simulink model "can8auto"  (R2018a)
settings: Solver=VariableStepAuto  StartTime=0.0  StopTime=5000  RelTol=1e-3
libraries: commcrc2 x20, simulink x20, simulink_extras x5, dspswit3 x5
(part 7 of 7)

== matlab function can8auto/CAN MASTER/MATLAB Function ==
  data: parallel input; serial output size=1; current_index input size=1; next_index output size=1; state input; endTX output
  events: trigger input RISING_EDGE_EVENT
function [serial,next_index,endTX] = parallelToSerial(parallel,current_index, state)
    size_parallel = size(parallel);
    size_parallel = size_parallel(2);
    endTX = 0;
    serial = 1;
    next_index = 1;
    if current_index < size_parallel && (state == 2 || state == 3)
        serial = parallel(current_index+1);
        next_index = current_index + 1;
        return
    end
    if current_index == size_parallel && (state == 2 || state == 3)
        endTX = 1;
    end
end

== matlab function can8auto/SDO NODO CAN/CAN NODE/SDO Frame generator/BitStuffing/MATLAB Function ==
  data: u input; b output
function b = fcn(u)
a = u;
b = zeros(1,floor(length(a)+length(a)/5));
k = 0;
count2 = 1;
i = 1;
n = length(a);
count = 1;
j = 1;
while i < n
    if a(i) == 1
        b(j) = a(i);
        while a(i+1) == 1 && i+1 < n && count < 5
            j = j+1;
            b(j) = a(i+1);
            count = count + 1;
            count2 = count;
            if count == 5
                j = j+1;
                b(j) = 0;
            end
            i = i+1;
        end
        
    else
        b(j) = a(i);
    end
    
    if a(i) == 0
    if a(i) == 0
        b(j) = a(i);
        while a(i+1) == 0 && i+1 < n && count < 5
            j = j+1;
            b(j) = a(i+1);
            count = count + 1;
            count2 = count;
            if count == 5
                j = j+1;
                b(j) = 1;
            end
            i = i+1;
        end
        
    else
        b(j) = a(i);
    end
    end
    
    i = i+1;
    j = j+1;
    count = 1;
end
if i == n && a(i) == 1 && count2 == 4
    b(j) = a(i);
    b(j+1) = 0;
else
    b(j) = a(i);
end

if i == n && a(i) == 0 && count2 == 4
    b(j) = a(i);
    b(j+1) = 1;
else
    b(j) = a(i);
end

== stateflow chart can8auto/SDO NODO CAN/SlaveSDO ==
  state BootUp
    entry: mode = 0;
  state NormalOp
    entry: mode = 2;
  (default) -> BootUp
  NormalOp -> BootUp : [rst == 1]
  BootUp -> NormalOp : [SDO == 1 && EndTX == 1 && TotTX == 2]
  data: rst input; SDO input; TotTX input; EndTX input; mode output

== matlab function can8auto/SYNC PRODUCER/CAN NODE/Bootup Frame generator/BitStuffing/MATLAB Function ==
  data: u input; b output
function b = fcn(u)
a = u;
b = zeros(1,floor(length(a)+length(a)/5));
k = 0;
count2 = 1;
i = 1;
n = length(a);
count = 1;
j = 1;
while i < n
    if a(i) == 1
        b(j) = a(i);
        while a(i+1) == 1 && i+1 < n && count < 5
            j = j+1;
            b(j) = a(i+1);
            count = count + 1;
            count2 = count;
            if count == 5
                j = j+1;
                b(j) = 0;
            end
            i = i+1;
        end
        
    else
        b(j) = a(i);
    end
    
    if a(i) == 0
    if a(i) == 0
        b(j) = a(i);
        while a(i+1) == 0 && i+1 < n && count < 5
            j = j+1;
            b(j) = a(i+1);
            count = count + 1;
            count2 = count;
            if count == 5
                j = j+1;
                b(j) = 1;
            end
            i = i+1;
        end
        
    else
        b(j) = a(i);
    end
    end
    
    i = i+1;
    j = j+1;
    count = 1;
end
if i == n && a(i) == 1 && count2 == 4
    b(j) = a(i);
    b(j+1) = 0;
else
    b(j) = a(i);
end

if i == n && a(i) == 0 && count2 == 4
    b(j) = a(i);
    b(j+1) = 1;
else
    b(j) = a(i);
end

== matlab function can8auto/SDO NODO CAN/CAN NODE/SDO Frame generator/MUX/MATLAB Function ==
  data: index input; result output size=[1 64]; u1 input
function result  = mux(index, u1)
%#codegen
%
% Insert zeros between elements

result = zeros(1,64);
switch index
    case 0
        result = u1(1:64);
    case 1
        result = u1(65:128);
    case 2
        result = u1(129:192);
    otherwise
        result = u1(193:256);
end

== matlab function can8auto/SYNC PRODUCER/MATLAB Function ==
  data: u input size=1; y output size=1
function y = equals4(u)
    if u == 4
        y = 1;
    else
        y = 0;
    end
end

== matlab function can8auto/SYNC PRODUCER/CAN NODE/Frame MUX/MATLAB Function2 ==
  data: mode input; result output size=[1 200]; u1 input; size input
function result = MUX_lv2(mode, u1, size)
%#codegen
%
% Insert zeros between elements

switch mode
    case 0
        result = u1(1 : size(1));
    case 1
        result = u1(size(1)+1 : size(1)+size(2));
    case 2
        result = u1(size(1)+size(2)+1 : size(1)+size(2)+size(3));
    case 3
        result = u1(size(1)+size(2)+size(3)+1 : size(1)+size(2)+size(3)+size(4));
    otherwise
        result = u1(size(1)+size(2)+size(3)+size(4)+1 : size(1)+size(2)+size(3)+size(4)+size(5));
end

== stateflow chart can8auto/CAN MASTER/Master ==
  state BootUp
    entry: sigOut = 0;
  state NMT
    entry: PDO = 1;
    entry: SDO = 1;
    entry: sigOut = 1;
  state NormalOp
    entry: sigOut = 2;
  (default) -> BootUp
  BootUp -> NMT : [EndTX == 1 && totalTX == 2]
  NormalOp -> BootUp : [rst == 1]
  NMT -> NormalOp : [EndTX == 1 && totalTX == 3]
  data: rst input; SDO output; PDO output; sigOut output; EndTX input; totalTX input

== matlab function can8auto/CAN MASTER/MATLAB Function1 ==
  data: u input size=1; y output size=1
function y = fcn(u)
if u == 1
    y = true;
else
    y = false;
end

== matlab function can8auto/SDO NODO CAN/CAN NODE/SYNC Frame Generator/BitStuffing/MATLAB Function ==
  data: u input; b output
function b = fcn(u)
a = u;
b = zeros(1,floor(length(a)+length(a)/5));
k = 0;
count2 = 1;
i = 1;
n = length(a);
count = 1;
j = 1;
while i < n
    if a(i) == 1
        b(j) = a(i);
        while a(i+1) == 1 && i+1 < n && count < 5
            j = j+1;
            b(j) = a(i+1);
            count = count + 1;
            count2 = count;
            if count == 5
                j = j+1;
                b(j) = 0;
            end
            i = i+1;
        end
        
    else
        b(j) = a(i);
    end
    
    if a(i) == 0
    if a(i) == 0
        b(j) = a(i);
        while a(i+1) == 0 && i+1 < n && count < 5
            j = j+1;
            b(j) = a(i+1);
            count = count + 1;
            count2 = count;
            if count == 5
                j = j+1;
                b(j) = 1;
            end
            i = i+1;
        end
        
    else
        b(j) = a(i);
    end
    end
    
    i = i+1;
    j = j+1;
    count = 1;
end
if i == n && a(i) == 1 && count2 == 4
    b(j) = a(i);
    b(j+1) = 0;
else
    b(j) = a(i);
end

if i == n && a(i) == 0 && count2 == 4
    b(j) = a(i);
    b(j+1) = 1;
else
    b(j) = a(i);
end

== stateflow chart can8auto/SDO NODO CAN/Chart ==
  state NoTX
    entry: state = 0;
  state SenseBus
    entry: state = 1;
  state TXcompleated
    entry: state = 4;
  state TX
    entry: state = 2;
  NoTX -> NoTX [order 2] : [Frame == 0]
  SenseBus -> SenseBus [order 1] : [Free == 0 || EndTX == 1]
  (default) -> NoTX
  TXcompleated -> NoTX [order 1] : [Frame == 0]
  NoTX -> SenseBus [order 1] : [Frame  > 0]
  TX -> SenseBus [order 2] : [Error == 1]
  TXcompleated -> SenseBus [order 2] : [Frame  > 0]
  SenseBus -> TX [order 2] : [Free == 1]
  TX -> TXcompleated [order 1] : [EndTX == 1]
  TX -> TX [order 3]
  data: Free input; Error input; Frame input; EndTX input; state output

== matlab function can8auto/SDO NODO CAN/MATLAB Function ==
  data: parallel input; serial output size=1; current_index input size=1; next_index output size=1; state input; endTX output
  events: trigger input RISING_EDGE_EVENT
function [serial,next_index,endTX] = parallelToSerial(parallel,current_index, state)
    size_parallel = size(parallel);
    size_parallel = size_parallel(2);
    endTX = 0;
    serial = 1;
    next_index = 1;
    if current_index < size_parallel && (state == 2 || state == 3)
        serial = parallel(current_index+1);
        next_index = current_index + 1;
        return
    end
    if current_index == size_parallel && (state == 2 || state == 3)
        endTX = 1;
    end
end

== matlab function can8auto/SDO NODO CAN/MATLAB Function1 ==
  data: u input size=1; y output size=1
function y = fcn(u)
if u == 1
    y = true;
else
    y = false;
end

== matlab function can8auto/SDO NODO CAN/Sensing/MATLAB Function ==
  data: BusState input; free output; clock input; count input; count output
  events: trigger input RISING_EDGE_EVENT
function [free, count] = fcn(BusState, clock, count)
if clock
    if BusState
        count = count + 1;
    else
        count = 0;
    end
end
if count >= 20
    free = 1;
else
    free = 0;
end

== matlab function can8auto/CAN MASTER/Sensing/MATLAB Function ==
  data: BusState input; free output; clock input; count input; count output
  events: trigger input RISING_EDGE_EVENT
function [free, count] = fcn(BusState, clock, count)
if clock
    if BusState
        count = count + 1;
    else
        count = 0;
    end
end
if count >= 20
    free = 1;
else
    free = 0;
end

== stateflow chart can8auto/PDO NODO CAN /SlavePDO ==
  state BootUp
    entry: mode = 0;
  state Normal
    entry: mode = 3;
  (default) -> BootUp
  Normal -> BootUp : [rst == 1]
  BootUp -> Normal : [PDO == 1 && EndTX == 1]
  data: rst input; PDO input; EndTX input; mode output

== matlab function can8auto/SYNC PRODUCER/CAN NODE/NMT Frame generator/BitStuffing/MATLAB Function ==
  data: u input; b output
function b = fcn(u)
a = u;
b = zeros(1,floor(length(a)+length(a)/5));
k = 0;
count2 = 1;
i = 1;
n = length(a);
count = 1;
j = 1;
while i < n
    if a(i) == 1
        b(j) = a(i);
        while a(i+1) == 1 && i+1 < n && count < 5
            j = j+1;
            b(j) = a(i+1);
            count = count + 1;
            count2 = count;
            if count == 5
                j = j+1;
                b(j) = 0;
            end
            i = i+1;
        end
        
    else
        b(j) = a(i);
    end
    
    if a(i) == 0
    if a(i) == 0
        b(j) = a(i);
        while a(i+1) == 0 && i+1 < n && count < 5
            j = j+1;
            b(j) = a(i+1);
            count = count + 1;
            count2 = count;
            if count == 5
                j = j+1;
                b(j) = 1;
            end
            i = i+1;
        end
        
    else
        b(j) = a(i);
    end
    end
    
    i = i+1;
    j = j+1;
    count = 1;
end
if i == n && a(i) == 1 && count2 == 4
    b(j) = a(i);
    b(j+1) = 0;
else
    b(j) = a(i);
end

if i == n && a(i) == 0 && count2 == 4
    b(j) = a(i);
    b(j+1) = 1;
else
    b(j) = a(i);
end

== matlab function can8auto/SYNC PRODUCER/CAN NODE/SDO Frame generator/BitStuffing/MATLAB Function ==
  data: u input; b output
function b = fcn(u)
a = u;
b = zeros(1,floor(length(a)+length(a)/5));
k = 0;
count2 = 1;
i = 1;
n = length(a);
count = 1;
j = 1;
while i < n
    if a(i) == 1
        b(j) = a(i);
        while a(i+1) == 1 && i+1 < n && count < 5
            j = j+1;
            b(j) = a(i+1);
            count = count + 1;
            count2 = count;
            if count == 5
                j = j+1;
                b(j) = 0;
            end
            i = i+1;
        end
        
    else
        b(j) = a(i);
    end
    
    if a(i) == 0
    if a(i) == 0
        b(j) = a(i);
        while a(i+1) == 0 && i+1 < n && count < 5
            j = j+1;
            b(j) = a(i+1);
            count = count + 1;
            count2 = count;
            if count == 5
                j = j+1;
                b(j) = 1;
            end
            i = i+1;
        end
        
    else
        b(j) = a(i);
    end
    end
    
    i = i+1;
    j = j+1;
    count = 1;
end
if i == n && a(i) == 1 && count2 == 4
    b(j) = a(i);
    b(j+1) = 0;
else
    b(j) = a(i);
end

if i == n && a(i) == 0 && count2 == 4
    b(j) = a(i);
    b(j+1) = 1;
else
    b(j) = a(i);
end

== matlab function can8auto/PDO NODO CAN /CAN NODE/Bootup Frame generator/BitStuffing/MATLAB Function ==
  data: u input; b output
function b = fcn(u)
a = u;
b = zeros(1,floor(length(a)+length(a)/5));
k = 0;
count2 = 1;
i = 1;
n = length(a);
count = 1;
j = 1;
while i < n
    if a(i) == 1
        b(j) = a(i);
        while a(i+1) == 1 && i+1 < n && count < 5
            j = j+1;
            b(j) = a(i+1);
            count = count + 1;
            count2 = count;
            if count == 5
                j = j+1;
                b(j) = 0;
            end
            i = i+1;
        end
        
    else
        b(j) = a(i);
    end
    
    if a(i) == 0
    if a(i) == 0
        b(j) = a(i);
        while a(i+1) == 0 && i+1 < n && count < 5
            j = j+1;
            b(j) = a(i+1);
            count = count + 1;
            count2 = count;
            if count == 5
                j = j+1;
                b(j) = 1;
            end
            i = i+1;
        end
        
    else
        b(j) = a(i);
    end
    end
    
    i = i+1;
    j = j+1;
    count = 1;
end
if i == n && a(i) == 1 && count2 == 4
    b(j) = a(i);
    b(j+1) = 0;
else
    b(j) = a(i);
end

if i == n && a(i) == 0 && count2 == 4
    b(j) = a(i);
    b(j+1) = 1;
else
    b(j) = a(i);
end

== matlab function can8auto/SYNC PRODUCER/CAN NODE/SDO Frame generator/MUX/MATLAB Function ==
  data: index input; result output size=[1 64]; u1 input
function result  = mux(index, u1)
%#codegen
%
% Insert zeros between elements

result = zeros(1,64);
switch index
    case 0
        result = u1(1:64);
    case 1
        result = u1(65:128);
    case 2
        result = u1(129:192);
    otherwise
        result = u1(193:256);
end

== matlab function can8auto/PDO NODO CAN /CAN NODE/Frame MUX/MATLAB Function2 ==
  data: mode input; result output size=[1 200]; u1 input; size input
function result = MUX_lv2(mode, u1, size)
%#codegen
%
% Insert zeros between elements

switch mode
    case 0
        result = u1(1 : size(1));
    case 1
        result = u1(size(1)+1 : size(1)+size(2));
    case 2
        result = u1(size(1)+size(2)+1 : size(1)+size(2)+size(3));
    case 3
        result = u1(size(1)+size(2)+size(3)+1 : size(1)+size(2)+size(3)+size(4));
    otherwise
        result = u1(size(1)+size(2)+size(3)+size(4)+1 : size(1)+size(2)+size(3)+size(4)+size(5));
end

== matlab function can8auto/PDO NODO CAN /CAN NODE/NMT Frame generator/BitStuffing/MATLAB Function ==
  data: u input; b output
function b = fcn(u)
a = u;
b = zeros(1,floor(length(a)+length(a)/5));
k = 0;
count2 = 1;
i = 1;
n = length(a);
count = 1;
j = 1;
while i < n
    if a(i) == 1
        b(j) = a(i);
        while a(i+1) == 1 && i+1 < n && count < 5
            j = j+1;
            b(j) = a(i+1);
            count = count + 1;
            count2 = count;
            if count == 5
                j = j+1;
                b(j) = 0;
            end
            i = i+1;
        end
        
    else
        b(j) = a(i);
    end
    
    if a(i) == 0
    if a(i) == 0
        b(j) = a(i);
        while a(i+1) == 0 && i+1 < n && count < 5
            j = j+1;
            b(j) = a(i+1);
            count = count + 1;
            count2 = count;
            if count == 5
                j = j+1;
                b(j) = 1;
            end
            i = i+1;
        end
        
    else
        b(j) = a(i);
    end
    end
    
    i = i+1;
    j = j+1;
    count = 1;
end
if i == n && a(i) == 1 && count2 == 4
    b(j) = a(i);
    b(j+1) = 0;
else
    b(j) = a(i);
end

if i == n && a(i) == 0 && count2 == 4
    b(j) = a(i);
    b(j+1) = 1;
else
    b(j) = a(i);
end

== matlab function can8auto/PDO NODO CAN /CAN NODE/SDO Frame generator/BitStuffing/MATLAB Function ==
  data: u input; b output
function b = fcn(u)
a = u;
b = zeros(1,floor(length(a)+length(a)/5));
k = 0;
count2 = 1;
i = 1;
n = length(a);
count = 1;
j = 1;
while i < n
    if a(i) == 1
        b(j) = a(i);
        while a(i+1) == 1 && i+1 < n && count < 5
            j = j+1;
            b(j) = a(i+1);
            count = count + 1;
            count2 = count;
            if count == 5
                j = j+1;
                b(j) = 0;
            end
            i = i+1;
        end
        
    else
        b(j) = a(i);
    end
    
    if a(i) == 0
    if a(i) == 0
        b(j) = a(i);
        while a(i+1) == 0 && i+1 < n && count < 5
            j = j+1;
            b(j) = a(i+1);
            count = count + 1;
            count2 = count;
            if count == 5
                j = j+1;
                b(j) = 1;
            end
            i = i+1;
        end
        
    else
        b(j) = a(i);
    end
    end
    
    i = i+1;
    j = j+1;
    count = 1;
end
if i == n && a(i) == 1 && count2 == 4
    b(j) = a(i);
    b(j+1) = 0;
else
    b(j) = a(i);
end

if i == n && a(i) == 0 && count2 == 4
    b(j) = a(i);
    b(j+1) = 1;
else
    b(j) = a(i);
end

== matlab function can8auto/PDO NODO CAN /CAN NODE/SDO Frame generator/MUX/MATLAB Function ==
  data: index input; result output size=[1 64]; u1 input
function result  = mux(index, u1)
%#codegen
%
% Insert zeros between elements

result = zeros(1,64);
switch index
    case 0
        result = u1(1:64);
    case 1
        result = u1(65:128);
    case 2
        result = u1(129:192);
    otherwise
        result = u1(193:256);
end

== matlab function can8auto/PDO NODO CAN /CAN NODE/SYNC Frame Generator/BitStuffing/MATLAB Function ==
  data: u input; b output
function b = fcn(u)
a = u;
b = zeros(1,floor(length(a)+length(a)/5));
k = 0;
count2 = 1;
i = 1;
n = length(a);
count = 1;
j = 1;
while i < n
    if a(i) == 1
        b(j) = a(i);
        while a(i+1) == 1 && i+1 < n && count < 5
            j = j+1;
            b(j) = a(i+1);
            count = count + 1;
            count2 = count;
            if count == 5
                j = j+1;
                b(j) = 0;
            end
            i = i+1;
        end
        
    else
        b(j) = a(i);
    end
    
    if a(i) == 0
    if a(i) == 0
        b(j) = a(i);
        while a(i+1) == 0 && i+1 < n && count < 5
            j = j+1;
            b(j) = a(i+1);
            count = count + 1;
            count2 = count;
            if count == 5
                j = j+1;
                b(j) = 1;
            end
            i = i+1;
        end
        
    else
        b(j) = a(i);
    end
    end
    
    i = i+1;
    j = j+1;
    count = 1;
end
if i == n && a(i) == 1 && count2 == 4
    b(j) = a(i);
    b(j+1) = 0;
else
    b(j) = a(i);
end

if i == n && a(i) == 0 && count2 == 4
    b(j) = a(i);
    b(j+1) = 1;
else
    b(j) = a(i);
end

== stateflow chart can8auto/PDO NODO CAN /Chart ==
  state NoTX
    entry: state = 0;
  state SenseBus
    entry: state = 1;
  state TXcompleated
    entry: state = 4;
  state TX
    entry: state = 2;
  NoTX -> NoTX [order 3] : [trigger == 0]
  SenseBus -> SenseBus [order 1] : [Free == 0]
  (default) -> NoTX
  NoTX -> SenseBus [order 1] : [trigger  > 0]
  TX -> SenseBus [order 2] : [Error == 1]
  TXcompleated -> NoTX [order 1] : [trigger == 0]
  NoTX -> SenseBus [order 2] : [mode == 0 && NewTX ==1]
  TXcompleated -> SenseBus [order 2] : [trigger  > 0]
  SenseBus -> TX [order 2] : [Free == 1]
  TX -> TX [order 3]
  TX -> TXcompleated [order 1] : [EndTX == 1]
  data: Free input; Error input; trigger input; EndTX input; state output; NewTX input; mode input

== matlab function can8auto/PDO NODO CAN /MATLAB Function ==
  data: parallel input; serial output size=1; current_index input size=1; next_index output size=1; state input; endTX output
  events: trigger input RISING_EDGE_EVENT
function [serial,next_index,endTX] = parallelToSerial(parallel,current_index, state)
    size_parallel = size(parallel);
    size_parallel = size_parallel(2);
    endTX = 0;
    serial = 1;
    next_index = 1;
    if current_index < size_parallel && (state == 2 || state == 3)
        serial = parallel(current_index+1);
        next_index = current_index + 1;
        return
    end
    if current_index == size_parallel && (state == 2 || state == 3)
        endTX = 1;
    end
end

== matlab function can8auto/PDO NODO CAN /MATLAB Function1 ==
  data: u input size=1; y output size=1
function y = fcn(u)
if u == 1
    y = true;
else
    y = false;
end

== matlab function can8auto/PDO NODO CAN /Sensing/MATLAB Function ==
  data: BusState input; free output; clock input; count input; count output
  events: trigger input RISING_EDGE_EVENT
function [free, count] = fcn(BusState, clock, count)
if clock
    if BusState
        count = count + 1;
    else
        count = 0;
    end
end
if count >= 20
    free = 1;
else
    free = 0;
end

== matlab function can8auto/SYNC PRODUCER/CAN NODE/SYNC Frame Generator/BitStuffing/MATLAB Function ==
  data: u input; b output
function b = fcn(u)
a = u;
b = zeros(1,floor(length(a)+length(a)/5));
k = 0;
count2 = 1;
i = 1;
n = length(a);
count = 1;
j = 1;
while i < n
    if a(i) == 1
        b(j) = a(i);
        while a(i+1) == 1 && i+1 < n && count < 5
            j = j+1;
            b(j) = a(i+1);
            count = count + 1;
            count2 = count;
            if count == 5
                j = j+1;
                b(j) = 0;
            end
            i = i+1;
        end
        
    else
        b(j) = a(i);
    end
    
    if a(i) == 0
    if a(i) == 0
        b(j) = a(i);
        while a(i+1) == 0 && i+1 < n && count < 5
            j = j+1;
            b(j) = a(i+1);
            count = count + 1;
            count2 = count;
            if count == 5
                j = j+1;
                b(j) = 1;
            end
            i = i+1;
        end
        
    else
        b(j) = a(i);
    end
    end
    
    i = i+1;
    j = j+1;
    count = 1;
end
if i == n && a(i) == 1 && count2 == 4
    b(j) = a(i);
    b(j+1) = 0;
else
    b(j) = a(i);
end

if i == n && a(i) == 0 && count2 == 4
    b(j) = a(i);
    b(j+1) = 1;
else
    b(j) = a(i);
end

== stateflow chart can8auto/SYNC PRODUCER/Chart ==
  state NoTX
    entry: state = 0;
  state SenseBus
    entry: state = 1;
  state TXcompleated
    entry: state = 4;
  state TX
    entry: state = 2;
  (default) -> NoTX
  SenseBus -> SenseBus [order 1] : [Free == 0]
  NoTX -> SenseBus [order 1] : [enableTX  > 0 && tempo == 1 ]
  NoTX -> SenseBus [order 2] : [mode == 0 && enableTX > 0]
  TX -> SenseBus [order 2] : [Error == 1]
  TXcompleated -> NoTX [order 2]
  TXcompleated -> SenseBus [order 1] : [enableTX  > 0 && tempo == 1 ]
  TXcompleated -> SenseBus [order 3] : [mode == 0 && enableTX > 0]
  SenseBus -> TX [order 2] : [Free == 1]
  TX -> TXcompleated [order 1] : [EndTX == 1]
  TX -> TX [order 3]
  data: Free input; Error input; EndTX input; state output; enableTX input; tempo input; mode input

== matlab function can8auto/SYNC PRODUCER/P//S converter ==
  data: parallel input; serial output size=1; current_index input size=1; next_index output size=1; state input; endTX output
  events: trigger input RISING_EDGE_EVENT
function [serial,next_index,endTX] = parallelToSerial(parallel,current_index, state)
    size_parallel = size(parallel);
    size_parallel = size_parallel(2);
    endTX = 0;
    serial = 1;
    next_index = 1;
    if current_index < size_parallel && (state == 2 || state == 3)
        serial = parallel(current_index+1);
        next_index = current_index + 1;
        return
    end
    if current_index == size_parallel && (state == 2 || state == 3)
        endTX = 1;
    end
end

== matlab function can8auto/SYNC PRODUCER/double to boolean ==
  data: u input size=1; y output size=1
function y = fcn(u)
if u == 1
    y = true;
else
    y = false;
end

== matlab function can8auto/SYNC PRODUCER/Sensing/MATLAB Function ==
  data: BusState input; free output; clock input; count input; count output
  events: trigger input RISING_EDGE_EVENT
function [free, count] = fcn(BusState, clock, count)
if clock
    if BusState
        count = count + 1;
    else
        count = 0;
    end
end
if count >= 20
    free = 1;
else
    free = 0;
end

== stateflow chart can8auto/SYNC PRODUCER/Chart1 ==
  state BootUp
    entry: mode = 0;
  state NormalOp
    entry: mode = 4;
  (default) -> BootUp
  BootUp -> NormalOp : [EndTX == 1]
  NormalOp -> BootUp [order 1] : [rst == 1]
  NormalOp -> NormalOp [order 2]
  data: EndTX input; rst input; mode output

== matlab function can8auto/PDO NODO CAN /Counter of Sync Messages/ADDER ==
  data: up input; val output; down input; counter input
  events: trigger1 input RISING_EDGE_EVENT
function val = counter(up, down, counter)
if (up == 1)
    counter = counter+1;
end
if (down == 1)
    counter = counter-1;
end
if(counter < 0)
    counter = 0;
end
val = counter;
